simulink model "pid"  (R2020b)
settings: Solver=VariableStepAuto  StartTime=0.0  StopTime=10.0  RelTol=1e-3
settings Model: Creator=shridhar  LastModifiedBy=shridhar

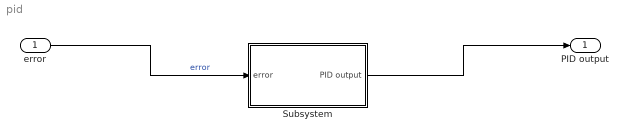
== system pid ==
  error : Inport  OutDataTypeStr=double  PortDimensions=1  SampleTime=0
  Subsystem : Subsystem
  PID output : Outport  OutDataTypeStr=double  PortDimensions=1  SampleTime=0
  wires:
  error/1 -> Subsystem/1(error)  "error"
  Subsystem/1(PID output) -> PID output/1

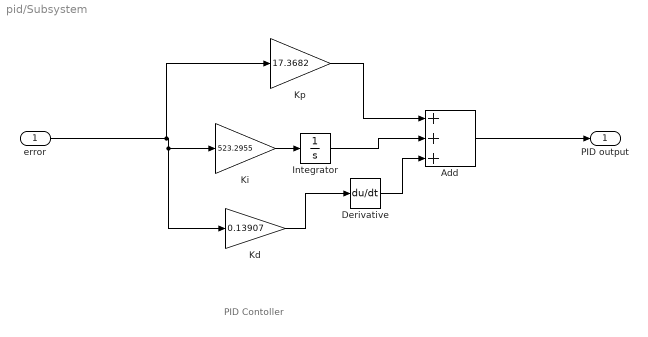
== system pid/Subsystem ==
  note: PID Contoller
  error : Inport  OutDataTypeStr=double  PortDimensions=1  SampleTime=0
  Add : Sum  Inputs=+++
  Derivative : Derivative
  Integrator : Integrator
  Kd : Gain  Gain=0.13907
  Ki : Gain  Gain=523.2955
  Kp : Gain  Gain=17.3682
  PID output : Outport  OutDataTypeStr=double  PortDimensions=1  SampleTime=0
  wires:
  Kd/1 -> Derivative/1
  Add/1 -> PID output/1
  Kp/1 -> Add/1
  error/1 -> Kp/1, Ki/1, Kd/1
  Integrator/1 -> Add/2
  Ki/1 -> Integrator/1
  Derivative/1 -> Add/3
